simulink model "original_decfir"  (R2012b)
settings: Solver=FixedStepDiscrete  SolverMode=SingleTasking  StartTime=0.0  StopTime=5000  FixedStep=1  RelTol=1e-3
libraries: xbsIndex_r4 x1499, xps_library x1, casper_library_misc x1
(part 7 of 15)

== system original_decfir/dec_fir/fir_dbl_col6 ==
  real1 : Inport
  imag1 : Inport  Port=2
  real2 : Inport  Port=3
  imag2 : Inport  Port=4
  real3 : Inport  Port=5
  imag3 : Inport  Port=6
  real4 : Inport  Port=7
  imag4 : Inport  Port=8
  real5 : Inport  Port=9
  imag5 : Inport  Port=10
  real6 : Inport  Port=11
  imag6 : Inport  Port=12
  real7 : Inport  Port=13
  imag7 : Inport  Port=14
  real8 : Inport  Port=15
  imag8 : Inport  Port=16
  real_back1 : Inport  Port=17
  imag_back1 : Inport  Port=18
  real_back2 : Inport  Port=19
  imag_back2 : Inport  Port=20
  real_back3 : Inport  Port=21
  imag_back3 : Inport  Port=22
  real_back4 : Inport  Port=23
  imag_back4 : Inport  Port=24
  real_back5 : Inport  Port=25
  imag_back5 : Inport  Port=26
  real_back6 : Inport  Port=27
  imag_back6 : Inport  Port=28
  real_back7 : Inport  Port=29
  imag_back7 : Inport  Port=30
  real_back8 : Inport  Port=31
  imag_back8 : Inport  Port=32
  adder_tree1 : Subsystem  AncestorBlock=casper_library_misc/adder_tree  mask(adder_tree){n_inputs=8, latency=1, adder_imp=Behavioral, first_stage_hdl=off}
      mask prompts: n_inputs "Number of Inputs"; latency "Add Latency"; adder_imp "Adder implementation"; first_stage_hdl "Use behavioural HDL for first stage of adders"
      mask help:
      | Sums all inputs using a tree of adds and delays.
      |
      | Number of inputs: The number of inputs to the block to be summed
      | Add latency: The number of clock cycles to perform one addition (affects timing)..
      | Adder implementation: choice of fabric or DSP48E core, or behavioral HDL
      | Use behavioural HDL for first stage of adders: Causes the first stage of adders to be absorbed into DSP blocks if multipliers precede them (Virtex 5). Overrides Adder implementation
      mask init:
      | adder_tree_init(gcb, ...
      |     'n_inputs', n_inputs, ...
      |     'latency', latency, ...
      |     'adder_imp', adder_imp, ...
      |     'first_stage_hdl', first_stage_hdl);
      settings: AttributesFormatString=latency 3
      mask Help: eval('xlWeb(''http://casper.berkeley.edu/wiki/Adder_tree'')')
      mask TypeOptions adder_imp: Behavioral | Fabric | DSP48
  adder_tree2 : Subsystem  AncestorBlock=casper_library_misc/adder_tree  mask(adder_tree){n_inputs=8, latency=1, adder_imp=Behavioral, first_stage_hdl=off}
      mask prompts: n_inputs "Number of Inputs"; latency "Add Latency"; adder_imp "Adder implementation"; first_stage_hdl "Use behavioural HDL for first stage of adders"
      mask help:
      | Sums all inputs using a tree of adds and delays.
      |
      | Number of inputs: The number of inputs to the block to be summed
      | Add latency: The number of clock cycles to perform one addition (affects timing)..
      | Adder implementation: choice of fabric or DSP48E core, or behavioral HDL
      | Use behavioural HDL for first stage of adders: Causes the first stage of adders to be absorbed into DSP blocks if multipliers precede them (Virtex 5). Overrides Adder implementation
      mask init:
      | adder_tree_init(gcb, ...
      |     'n_inputs', n_inputs, ...
      |     'latency', latency, ...
      |     'adder_imp', adder_imp, ...
      |     'first_stage_hdl', first_stage_hdl);
      settings: AttributesFormatString=latency 3
      mask Help: eval('xlWeb(''http://casper.berkeley.edu/wiki/Adder_tree'')')
      mask TypeOptions adder_imp: Behavioral | Fabric | DSP48
  c1 : xbsIndex_r4/Constant  const=1  gui_display_data_type=Fixed-point  arith_type=Signed (2's comp)  n_bits=16  bin_pt=14  preci_type=Single  exp_width=8  frac_width=24  explicit_period=on  period=1  equ=P=C  opselect=C  inp2=PCIN>>17  opr=+  inp1=P  carry=CIN  dbl_ovrd=off  block_type=constant
  c2 : xbsIndex_r4/Constant  const=1  gui_display_data_type=Fixed-point  arith_type=Signed (2's comp)  n_bits=16  bin_pt=14  preci_type=Single  exp_width=8  frac_width=24  explicit_period=on  period=1  equ=P=C  opselect=C  inp2=PCIN>>17  opr=+  inp1=P  carry=CIN  dbl_ovrd=off  block_type=constant
  fir_dbl_tap1 : Subsystem  AncestorBlock=casper_library_downconverter/fir_dbl_tap  mask(fir_dbl_tap){factor=-0.0012722, add_latency=add_latency, mult_latency=mult_latency, coeff_bit_width=coeff_bit_width, coeff_bin_pt=coeff_bin_pt}
      mask prompts: add_latency "Add latency"; mult_latency "Mult latency"; coeff_bit_width "Coefficient bit width"; coeff_bin_pt "Coefficient binary point"
      mask init: same as original_decfir/dec_fir/fir_dbl_col1/fir_dbl_tap1
      mask Help: eval('xlWeb(''http://casper.berkeley.edu/wiki/Fir_dbl_tap'')')
  fir_dbl_tap2 : Subsystem  AncestorBlock=casper_library_downconverter/fir_dbl_tap  mask(fir_dbl_tap){factor=-0.0012742, add_latency=add_latency, mult_latency=mult_latency, coeff_bit_width=coeff_bit_width, coeff_bin_pt=coeff_bin_pt}
      mask prompts: add_latency "Add latency"; mult_latency "Mult latency"; coeff_bit_width "Coefficient bit width"; coeff_bin_pt "Coefficient binary point"
      mask init: same as original_decfir/dec_fir/fir_dbl_col1/fir_dbl_tap1
      mask Help: eval('xlWeb(''http://casper.berkeley.edu/wiki/Fir_dbl_tap'')')
  fir_dbl_tap3 : Subsystem  AncestorBlock=casper_library_downconverter/fir_dbl_tap  mask(fir_dbl_tap){factor=-0.0011107, add_latency=add_latency, mult_latency=mult_latency, coeff_bit_width=coeff_bit_width, coeff_bin_pt=coeff_bin_pt}
      mask prompts: add_latency "Add latency"; mult_latency "Mult latency"; coeff_bit_width "Coefficient bit width"; coeff_bin_pt "Coefficient binary point"
      mask init: same as original_decfir/dec_fir/fir_dbl_col1/fir_dbl_tap1
      mask Help: eval('xlWeb(''http://casper.berkeley.edu/wiki/Fir_dbl_tap'')')
  fir_dbl_tap4 : Subsystem  AncestorBlock=casper_library_downconverter/fir_dbl_tap  mask(fir_dbl_tap){factor=-0.00081658, add_latency=add_latency, mult_latency=mult_latency, coeff_bit_width=coeff_bit_width, coeff_bin_pt=coeff_bin_pt}
      mask prompts: add_latency "Add latency"; mult_latency "Mult latency"; coeff_bit_width "Coefficient bit width"; coeff_bin_pt "Coefficient binary point"
      mask init: same as original_decfir/dec_fir/fir_dbl_col1/fir_dbl_tap1
      mask Help: eval('xlWeb(''http://casper.berkeley.edu/wiki/Fir_dbl_tap'')')
  fir_dbl_tap5 : Subsystem  AncestorBlock=casper_library_downconverter/fir_dbl_tap  mask(fir_dbl_tap){factor=-0.0004409, add_latency=add_latency, mult_latency=mult_latency, coeff_bit_width=coeff_bit_width, coeff_bin_pt=coeff_bin_pt}
      mask prompts: add_latency "Add latency"; mult_latency "Mult latency"; coeff_bit_width "Coefficient bit width"; coeff_bin_pt "Coefficient binary point"
      mask init: same as original_decfir/dec_fir/fir_dbl_col1/fir_dbl_tap1
      mask Help: eval('xlWeb(''http://casper.berkeley.edu/wiki/Fir_dbl_tap'')')
  fir_dbl_tap6 : Subsystem  AncestorBlock=casper_library_downconverter/fir_dbl_tap  mask(fir_dbl_tap){factor=-3.9415e-05, add_latency=add_latency, mult_latency=mult_latency, coeff_bit_width=coeff_bit_width, coeff_bin_pt=coeff_bin_pt}
      mask prompts: add_latency "Add latency"; mult_latency "Mult latency"; coeff_bit_width "Coefficient bit width"; coeff_bin_pt "Coefficient binary point"
      mask init: same as original_decfir/dec_fir/fir_dbl_col1/fir_dbl_tap1
      mask Help: eval('xlWeb(''http://casper.berkeley.edu/wiki/Fir_dbl_tap'')')
  fir_dbl_tap7 : Subsystem  AncestorBlock=casper_library_downconverter/fir_dbl_tap  mask(fir_dbl_tap){factor=0.00033331, add_latency=add_latency, mult_latency=mult_latency, coeff_bit_width=coeff_bit_width, coeff_bin_pt=coeff_bin_pt}
      mask prompts: add_latency "Add latency"; mult_latency "Mult latency"; coeff_bit_width "Coefficient bit width"; coeff_bin_pt "Coefficient binary point"
      mask init: same as original_decfir/dec_fir/fir_dbl_col1/fir_dbl_tap1
      mask Help: eval('xlWeb(''http://casper.berkeley.edu/wiki/Fir_dbl_tap'')')
  fir_dbl_tap8 : Subsystem  AncestorBlock=casper_library_downconverter/fir_dbl_tap  mask(fir_dbl_tap){factor=0.00063107, add_latency=add_latency, mult_latency=mult_latency, coeff_bit_width=coeff_bit_width, coeff_bin_pt=coeff_bin_pt}
      mask prompts: add_latency "Add latency"; mult_latency "Mult latency"; coeff_bit_width "Coefficient bit width"; coeff_bin_pt "Coefficient binary point"
      mask init: same as original_decfir/dec_fir/fir_dbl_col1/fir_dbl_tap1
      mask Help: eval('xlWeb(''http://casper.berkeley.edu/wiki/Fir_dbl_tap'')')
  term1 : Terminator
  term2 : Terminator
  real_out1 : Outport
  imag_out1 : Outport  Port=2
  real_out2 : Outport  Port=3
  imag_out2 : Outport  Port=4
  real_out3 : Outport  Port=5
  imag_out3 : Outport  Port=6
  real_out4 : Outport  Port=7
  imag_out4 : Outport  Port=8
  real_out5 : Outport  Port=9
  imag_out5 : Outport  Port=10
  real_out6 : Outport  Port=11
  imag_out6 : Outport  Port=12
  real_out7 : Outport  Port=13
  imag_out7 : Outport  Port=14
  real_out8 : Outport  Port=15
  imag_out8 : Outport  Port=16
  real_back_out1 : Outport  Port=17
  imag_back_out1 : Outport  Port=18
  real_back_out2 : Outport  Port=19
  imag_back_out2 : Outport  Port=20
  real_back_out3 : Outport  Port=21
  imag_back_out3 : Outport  Port=22
  real_back_out4 : Outport  Port=23
  imag_back_out4 : Outport  Port=24
  real_back_out5 : Outport  Port=25
  imag_back_out5 : Outport  Port=26
  real_back_out6 : Outport  Port=27
  imag_back_out6 : Outport  Port=28
  real_back_out7 : Outport  Port=29
  imag_back_out7 : Outport  Port=30
  real_back_out8 : Outport  Port=31
  imag_back_out8 : Outport  Port=32
  real_sum : Outport  Port=33
  imag_sum : Outport  Port=34
  wires:
  adder_tree1/1(sync_out) -> term1/1
  adder_tree2/1(sync_out) -> term2/1
  c1/1 -> adder_tree1/1(sync)
  c2/1 -> adder_tree2/1(sync)
  adder_tree1/2(dout) -> real_sum/1
  adder_tree2/2(dout) -> imag_sum/1
  real1/1 -> fir_dbl_tap1/1(a)
  imag1/1 -> fir_dbl_tap1/2(b)
  real_back8/1 -> fir_dbl_tap1/3(c)
  imag_back8/1 -> fir_dbl_tap1/4(d)
  fir_dbl_tap1/1(a_out) -> real_out1/1
  fir_dbl_tap1/2(b_out) -> imag_out1/1
  fir_dbl_tap1/3(c_out) -> real_back_out8/1
  fir_dbl_tap1/4(d_out) -> imag_back_out8/1
  fir_dbl_tap1/5(real) -> adder_tree1/2(din1)
  fir_dbl_tap1/6(imag) -> adder_tree2/2(din1)
  real2/1 -> fir_dbl_tap2/1(a)
  imag2/1 -> fir_dbl_tap2/2(b)
  real_back7/1 -> fir_dbl_tap2/3(c)
  imag_back7/1 -> fir_dbl_tap2/4(d)
  fir_dbl_tap2/1(a_out) -> real_out2/1
  fir_dbl_tap2/2(b_out) -> imag_out2/1
  fir_dbl_tap2/3(c_out) -> real_back_out7/1
  fir_dbl_tap2/4(d_out) -> imag_back_out7/1
  fir_dbl_tap2/5(real) -> adder_tree1/3(din2)
  fir_dbl_tap2/6(imag) -> adder_tree2/3(din2)
  real3/1 -> fir_dbl_tap3/1(a)
  imag3/1 -> fir_dbl_tap3/2(b)
  real_back6/1 -> fir_dbl_tap3/3(c)
  imag_back6/1 -> fir_dbl_tap3/4(d)
  fir_dbl_tap3/1(a_out) -> real_out3/1
  fir_dbl_tap3/2(b_out) -> imag_out3/1
  fir_dbl_tap3/3(c_out) -> real_back_out6/1
  fir_dbl_tap3/4(d_out) -> imag_back_out6/1
  fir_dbl_tap3/5(real) -> adder_tree1/4(din3)
  fir_dbl_tap3/6(imag) -> adder_tree2/4(din3)
  real4/1 -> fir_dbl_tap4/1(a)
  imag4/1 -> fir_dbl_tap4/2(b)
  real_back5/1 -> fir_dbl_tap4/3(c)
  imag_back5/1 -> fir_dbl_tap4/4(d)
  fir_dbl_tap4/1(a_out) -> real_out4/1
  fir_dbl_tap4/2(b_out) -> imag_out4/1
  fir_dbl_tap4/3(c_out) -> real_back_out5/1
  fir_dbl_tap4/4(d_out) -> imag_back_out5/1
  fir_dbl_tap4/5(real) -> adder_tree1/5(din4)
  fir_dbl_tap4/6(imag) -> adder_tree2/5(din4)
  real5/1 -> fir_dbl_tap5/1(a)
  imag5/1 -> fir_dbl_tap5/2(b)
  real_back4/1 -> fir_dbl_tap5/3(c)
  imag_back4/1 -> fir_dbl_tap5/4(d)
  fir_dbl_tap5/1(a_out) -> real_out5/1
  fir_dbl_tap5/2(b_out) -> imag_out5/1
  fir_dbl_tap5/3(c_out) -> real_back_out4/1
  fir_dbl_tap5/4(d_out) -> imag_back_out4/1
  fir_dbl_tap5/5(real) -> adder_tree1/6(din5)
  fir_dbl_tap5/6(imag) -> adder_tree2/6(din5)
  real6/1 -> fir_dbl_tap6/1(a)
  imag6/1 -> fir_dbl_tap6/2(b)
  real_back3/1 -> fir_dbl_tap6/3(c)
  imag_back3/1 -> fir_dbl_tap6/4(d)
  fir_dbl_tap6/1(a_out) -> real_out6/1
  fir_dbl_tap6/2(b_out) -> imag_out6/1
  fir_dbl_tap6/3(c_out) -> real_back_out3/1
  fir_dbl_tap6/4(d_out) -> imag_back_out3/1
  fir_dbl_tap6/5(real) -> adder_tree1/7(din6)
  fir_dbl_tap6/6(imag) -> adder_tree2/7(din6)
  real7/1 -> fir_dbl_tap7/1(a)
  imag7/1 -> fir_dbl_tap7/2(b)
  real_back2/1 -> fir_dbl_tap7/3(c)
  imag_back2/1 -> fir_dbl_tap7/4(d)
  fir_dbl_tap7/1(a_out) -> real_out7/1
  fir_dbl_tap7/2(b_out) -> imag_out7/1
  fir_dbl_tap7/3(c_out) -> real_back_out2/1
  fir_dbl_tap7/4(d_out) -> imag_back_out2/1
  fir_dbl_tap7/5(real) -> adder_tree1/8(din7)
  fir_dbl_tap7/6(imag) -> adder_tree2/8(din7)
  real8/1 -> fir_dbl_tap8/1(a)
  imag8/1 -> fir_dbl_tap8/2(b)
  real_back1/1 -> fir_dbl_tap8/3(c)
  imag_back1/1 -> fir_dbl_tap8/4(d)
  fir_dbl_tap8/1(a_out) -> real_out8/1
  fir_dbl_tap8/2(b_out) -> imag_out8/1
  fir_dbl_tap8/3(c_out) -> real_back_out1/1
  fir_dbl_tap8/4(d_out) -> imag_back_out1/1
  fir_dbl_tap8/5(real) -> adder_tree1/9(din8)
  fir_dbl_tap8/6(imag) -> adder_tree2/9(din8)

== system original_decfir/dec_fir/fir_dbl_col7 ==
  real1 : Inport
  imag1 : Inport  Port=2
  real2 : Inport  Port=3
  imag2 : Inport  Port=4
  real3 : Inport  Port=5
  imag3 : Inport  Port=6
  real4 : Inport  Port=7
  imag4 : Inport  Port=8
  real5 : Inport  Port=9
  imag5 : Inport  Port=10
  real6 : Inport  Port=11
  imag6 : Inport  Port=12
  real7 : Inport  Port=13
  imag7 : Inport  Port=14
  real8 : Inport  Port=15
  imag8 : Inport  Port=16
  real_back1 : Inport  Port=17
  imag_back1 : Inport  Port=18
  real_back2 : Inport  Port=19
  imag_back2 : Inport  Port=20
  real_back3 : Inport  Port=21
  imag_back3 : Inport  Port=22
  real_back4 : Inport  Port=23
  imag_back4 : Inport  Port=24
  real_back5 : Inport  Port=25
  imag_back5 : Inport  Port=26
  real_back6 : Inport  Port=27
  imag_back6 : Inport  Port=28
  real_back7 : Inport  Port=29
  imag_back7 : Inport  Port=30
  real_back8 : Inport  Port=31
  imag_back8 : Inport  Port=32
  adder_tree1 : Subsystem  AncestorBlock=casper_library_misc/adder_tree  mask(adder_tree){n_inputs=8, latency=1, adder_imp=Behavioral, first_stage_hdl=off}
      mask prompts: n_inputs "Number of Inputs"; latency "Add Latency"; adder_imp "Adder implementation"; first_stage_hdl "Use behavioural HDL for first stage of adders"
      mask help:
      | Sums all inputs using a tree of adds and delays.
      |
      | Number of inputs: The number of inputs to the block to be summed
      | Add latency: The number of clock cycles to perform one addition (affects timing)..
      | Adder implementation: choice of fabric or DSP48E core, or behavioral HDL
      | Use behavioural HDL for first stage of adders: Causes the first stage of adders to be absorbed into DSP blocks if multipliers precede them (Virtex 5). Overrides Adder implementation
      mask init:
      | adder_tree_init(gcb, ...
      |     'n_inputs', n_inputs, ...
      |     'latency', latency, ...
      |     'adder_imp', adder_imp, ...
      |     'first_stage_hdl', first_stage_hdl);
      settings: AttributesFormatString=latency 3
      mask Help: eval('xlWeb(''http://casper.berkeley.edu/wiki/Adder_tree'')')
      mask TypeOptions adder_imp: Behavioral | Fabric | DSP48
  adder_tree2 : Subsystem  AncestorBlock=casper_library_misc/adder_tree  mask(adder_tree){n_inputs=8, latency=1, adder_imp=Behavioral, first_stage_hdl=off}
      mask prompts: n_inputs "Number of Inputs"; latency "Add Latency"; adder_imp "Adder implementation"; first_stage_hdl "Use behavioural HDL for first stage of adders"
      mask help:
      | Sums all inputs using a tree of adds and delays.
      |
      | Number of inputs: The number of inputs to the block to be summed
      | Add latency: The number of clock cycles to perform one addition (affects timing)..
      | Adder implementation: choice of fabric or DSP48E core, or behavioral HDL
      | Use behavioural HDL for first stage of adders: Causes the first stage of adders to be absorbed into DSP blocks if multipliers precede them (Virtex 5). Overrides Adder implementation
      mask init:
      | adder_tree_init(gcb, ...
      |     'n_inputs', n_inputs, ...
      |     'latency', latency, ...
      |     'adder_imp', adder_imp, ...
      |     'first_stage_hdl', first_stage_hdl);
      settings: AttributesFormatString=latency 3
      mask Help: eval('xlWeb(''http://casper.berkeley.edu/wiki/Adder_tree'')')
      mask TypeOptions adder_imp: Behavioral | Fabric | DSP48
  c1 : xbsIndex_r4/Constant  const=1  gui_display_data_type=Fixed-point  arith_type=Signed (2's comp)  n_bits=16  bin_pt=14  preci_type=Single  exp_width=8  frac_width=24  explicit_period=on  period=1  equ=P=C  opselect=C  inp2=PCIN>>17  opr=+  inp1=P  carry=CIN  dbl_ovrd=off  block_type=constant
  c2 : xbsIndex_r4/Constant  const=1  gui_display_data_type=Fixed-point  arith_type=Signed (2's comp)  n_bits=16  bin_pt=14  preci_type=Single  exp_width=8  frac_width=24  explicit_period=on  period=1  equ=P=C  opselect=C  inp2=PCIN>>17  opr=+  inp1=P  carry=CIN  dbl_ovrd=off  block_type=constant
  fir_dbl_tap1 : Subsystem  AncestorBlock=casper_library_downconverter/fir_dbl_tap  mask(fir_dbl_tap){factor=0.0018361, add_latency=add_latency, mult_latency=mult_latency, coeff_bit_width=coeff_bit_width, coeff_bin_pt=coeff_bin_pt}
      mask prompts: add_latency "Add latency"; mult_latency "Mult latency"; coeff_bit_width "Coefficient bit width"; coeff_bin_pt "Coefficient binary point"
      mask init: same as original_decfir/dec_fir/fir_dbl_col1/fir_dbl_tap1
      mask Help: eval('xlWeb(''http://casper.berkeley.edu/wiki/Fir_dbl_tap'')')
  fir_dbl_tap2 : Subsystem  AncestorBlock=casper_library_downconverter/fir_dbl_tap  mask(fir_dbl_tap){factor=0.0017079, add_latency=add_latency, mult_latency=mult_latency, coeff_bit_width=coeff_bit_width, coeff_bin_pt=coeff_bin_pt}
      mask prompts: add_latency "Add latency"; mult_latency "Mult latency"; coeff_bit_width "Coefficient bit width"; coeff_bin_pt "Coefficient binary point"
      mask init: same as original_decfir/dec_fir/fir_dbl_col1/fir_dbl_tap1
      mask Help: eval('xlWeb(''http://casper.berkeley.edu/wiki/Fir_dbl_tap'')')
  fir_dbl_tap3 : Subsystem  AncestorBlock=casper_library_downconverter/fir_dbl_tap  mask(fir_dbl_tap){factor=0.0013679, add_latency=add_latency, mult_latency=mult_latency, coeff_bit_width=coeff_bit_width, coeff_bin_pt=coeff_bin_pt}
      mask prompts: add_latency "Add latency"; mult_latency "Mult latency"; coeff_bit_width "Coefficient bit width"; coeff_bin_pt "Coefficient binary point"
      mask init: same as original_decfir/dec_fir/fir_dbl_col1/fir_dbl_tap1
      mask Help: eval('xlWeb(''http://casper.berkeley.edu/wiki/Fir_dbl_tap'')')
  fir_dbl_tap4 : Subsystem  AncestorBlock=casper_library_downconverter/fir_dbl_tap  mask(fir_dbl_tap){factor=0.00087646, add_latency=add_latency, mult_latency=mult_latency, coeff_bit_width=coeff_bit_width, coeff_bin_pt=coeff_bin_pt}
      mask prompts: add_latency "Add latency"; mult_latency "Mult latency"; coeff_bit_width "Coefficient bit width"; coeff_bin_pt "Coefficient binary point"
      mask init: same as original_decfir/dec_fir/fir_dbl_col1/fir_dbl_tap1
      mask Help: eval('xlWeb(''http://casper.berkeley.edu/wiki/Fir_dbl_tap'')')
  fir_dbl_tap5 : Subsystem  AncestorBlock=casper_library_downconverter/fir_dbl_tap  mask(fir_dbl_tap){factor=0.00030942, add_latency=add_latency, mult_latency=mult_latency, coeff_bit_width=coeff_bit_width, coeff_bin_pt=coeff_bin_pt}
      mask prompts: add_latency "Add latency"; mult_latency "Mult latency"; coeff_bit_width "Coefficient bit width"; coeff_bin_pt "Coefficient binary point"
      mask init: same as original_decfir/dec_fir/fir_dbl_col1/fir_dbl_tap1
      mask Help: eval('xlWeb(''http://casper.berkeley.edu/wiki/Fir_dbl_tap'')')
  fir_dbl_tap6 : Subsystem  AncestorBlock=casper_library_downconverter/fir_dbl_tap  mask(fir_dbl_tap){factor=-0.00025349, add_latency=add_latency, mult_latency=mult_latency, coeff_bit_width=coeff_bit_width, coeff_bin_pt=coeff_bin_pt}
      mask prompts: add_latency "Add latency"; mult_latency "Mult latency"; coeff_bit_width "Coefficient bit width"; coeff_bin_pt "Coefficient binary point"
      mask init: same as original_decfir/dec_fir/fir_dbl_col1/fir_dbl_tap1
      mask Help: eval('xlWeb(''http://casper.berkeley.edu/wiki/Fir_dbl_tap'')')
  fir_dbl_tap7 : Subsystem  AncestorBlock=casper_library_downconverter/fir_dbl_tap  mask(fir_dbl_tap){factor=-0.0007392, add_latency=add_latency, mult_latency=mult_latency, coeff_bit_width=coeff_bit_width, coeff_bin_pt=coeff_bin_pt}
      mask prompts: add_latency "Add latency"; mult_latency "Mult latency"; coeff_bit_width "Coefficient bit width"; coeff_bin_pt "Coefficient binary point"
      mask init: same as original_decfir/dec_fir/fir_dbl_col1/fir_dbl_tap1
      mask Help: eval('xlWeb(''http://casper.berkeley.edu/wiki/Fir_dbl_tap'')')
  fir_dbl_tap8 : Subsystem  AncestorBlock=casper_library_downconverter/fir_dbl_tap  mask(fir_dbl_tap){factor=-0.0010905, add_latency=add_latency, mult_latency=mult_latency, coeff_bit_width=coeff_bit_width, coeff_bin_pt=coeff_bin_pt}
      mask prompts: add_latency "Add latency"; mult_latency "Mult latency"; coeff_bit_width "Coefficient bit width"; coeff_bin_pt "Coefficient binary point"
      mask init: same as original_decfir/dec_fir/fir_dbl_col1/fir_dbl_tap1
      mask Help: eval('xlWeb(''http://casper.berkeley.edu/wiki/Fir_dbl_tap'')')
  term1 : Terminator
  term2 : Terminator
  real_out1 : Outport
  imag_out1 : Outport  Port=2
  real_out2 : Outport  Port=3
  imag_out2 : Outport  Port=4
  real_out3 : Outport  Port=5
  imag_out3 : Outport  Port=6
  real_out4 : Outport  Port=7
  imag_out4 : Outport  Port=8
  real_out5 : Outport  Port=9
  imag_out5 : Outport  Port=10
  real_out6 : Outport  Port=11
  imag_out6 : Outport  Port=12
  real_out7 : Outport  Port=13
  imag_out7 : Outport  Port=14
  real_out8 : Outport  Port=15
  imag_out8 : Outport  Port=16
  real_back_out1 : Outport  Port=17
  imag_back_out1 : Outport  Port=18
  real_back_out2 : Outport  Port=19
  imag_back_out2 : Outport  Port=20
  real_back_out3 : Outport  Port=21
  imag_back_out3 : Outport  Port=22
  real_back_out4 : Outport  Port=23
  imag_back_out4 : Outport  Port=24
  real_back_out5 : Outport  Port=25
  imag_back_out5 : Outport  Port=26
  real_back_out6 : Outport  Port=27
  imag_back_out6 : Outport  Port=28
  real_back_out7 : Outport  Port=29
  imag_back_out7 : Outport  Port=30
  real_back_out8 : Outport  Port=31
  imag_back_out8 : Outport  Port=32
  real_sum : Outport  Port=33
  imag_sum : Outport  Port=34
  wires:
  adder_tree1/1(sync_out) -> term1/1
  adder_tree2/1(sync_out) -> term2/1
  c1/1 -> adder_tree1/1(sync)
  c2/1 -> adder_tree2/1(sync)
  adder_tree1/2(dout) -> real_sum/1
  adder_tree2/2(dout) -> imag_sum/1
  real1/1 -> fir_dbl_tap1/1(a)
  imag1/1 -> fir_dbl_tap1/2(b)
  real_back8/1 -> fir_dbl_tap1/3(c)
  imag_back8/1 -> fir_dbl_tap1/4(d)
  fir_dbl_tap1/1(a_out) -> real_out1/1
  fir_dbl_tap1/2(b_out) -> imag_out1/1
  fir_dbl_tap1/3(c_out) -> real_back_out8/1
  fir_dbl_tap1/4(d_out) -> imag_back_out8/1
  fir_dbl_tap1/5(real) -> adder_tree1/2(din1)
  fir_dbl_tap1/6(imag) -> adder_tree2/2(din1)
  real2/1 -> fir_dbl_tap2/1(a)
  imag2/1 -> fir_dbl_tap2/2(b)
  real_back7/1 -> fir_dbl_tap2/3(c)
  imag_back7/1 -> fir_dbl_tap2/4(d)
  fir_dbl_tap2/1(a_out) -> real_out2/1
  fir_dbl_tap2/2(b_out) -> imag_out2/1
  fir_dbl_tap2/3(c_out) -> real_back_out7/1
  fir_dbl_tap2/4(d_out) -> imag_back_out7/1
  fir_dbl_tap2/5(real) -> adder_tree1/3(din2)
  fir_dbl_tap2/6(imag) -> adder_tree2/3(din2)
  real3/1 -> fir_dbl_tap3/1(a)
  imag3/1 -> fir_dbl_tap3/2(b)
  real_back6/1 -> fir_dbl_tap3/3(c)
  imag_back6/1 -> fir_dbl_tap3/4(d)
  fir_dbl_tap3/1(a_out) -> real_out3/1
  fir_dbl_tap3/2(b_out) -> imag_out3/1
  fir_dbl_tap3/3(c_out) -> real_back_out6/1
  fir_dbl_tap3/4(d_out) -> imag_back_out6/1
  fir_dbl_tap3/5(real) -> adder_tree1/4(din3)
  fir_dbl_tap3/6(imag) -> adder_tree2/4(din3)
  real4/1 -> fir_dbl_tap4/1(a)
  imag4/1 -> fir_dbl_tap4/2(b)
  real_back5/1 -> fir_dbl_tap4/3(c)
  imag_back5/1 -> fir_dbl_tap4/4(d)
  fir_dbl_tap4/1(a_out) -> real_out4/1
  fir_dbl_tap4/2(b_out) -> imag_out4/1
  fir_dbl_tap4/3(c_out) -> real_back_out5/1
  fir_dbl_tap4/4(d_out) -> imag_back_out5/1
  fir_dbl_tap4/5(real) -> adder_tree1/5(din4)
  fir_dbl_tap4/6(imag) -> adder_tree2/5(din4)
  real5/1 -> fir_dbl_tap5/1(a)
  imag5/1 -> fir_dbl_tap5/2(b)
  real_back4/1 -> fir_dbl_tap5/3(c)
  imag_back4/1 -> fir_dbl_tap5/4(d)
  fir_dbl_tap5/1(a_out) -> real_out5/1
  fir_dbl_tap5/2(b_out) -> imag_out5/1
  fir_dbl_tap5/3(c_out) -> real_back_out4/1
  fir_dbl_tap5/4(d_out) -> imag_back_out4/1
  fir_dbl_tap5/5(real) -> adder_tree1/6(din5)
  fir_dbl_tap5/6(imag) -> adder_tree2/6(din5)
  real6/1 -> fir_dbl_tap6/1(a)
  imag6/1 -> fir_dbl_tap6/2(b)
  real_back3/1 -> fir_dbl_tap6/3(c)
  imag_back3/1 -> fir_dbl_tap6/4(d)
  fir_dbl_tap6/1(a_out) -> real_out6/1
  fir_dbl_tap6/2(b_out) -> imag_out6/1
  fir_dbl_tap6/3(c_out) -> real_back_out3/1
  fir_dbl_tap6/4(d_out) -> imag_back_out3/1
  fir_dbl_tap6/5(real) -> adder_tree1/7(din6)
  fir_dbl_tap6/6(imag) -> adder_tree2/7(din6)
  real7/1 -> fir_dbl_tap7/1(a)
  imag7/1 -> fir_dbl_tap7/2(b)
  real_back2/1 -> fir_dbl_tap7/3(c)
  imag_back2/1 -> fir_dbl_tap7/4(d)
  fir_dbl_tap7/1(a_out) -> real_out7/1
  fir_dbl_tap7/2(b_out) -> imag_out7/1
  fir_dbl_tap7/3(c_out) -> real_back_out2/1
  fir_dbl_tap7/4(d_out) -> imag_back_out2/1
  fir_dbl_tap7/5(real) -> adder_tree1/8(din7)
  fir_dbl_tap7/6(imag) -> adder_tree2/8(din7)
  real8/1 -> fir_dbl_tap8/1(a)
  imag8/1 -> fir_dbl_tap8/2(b)
  real_back1/1 -> fir_dbl_tap8/3(c)
  imag_back1/1 -> fir_dbl_tap8/4(d)
  fir_dbl_tap8/1(a_out) -> real_out8/1
  fir_dbl_tap8/2(b_out) -> imag_out8/1
  fir_dbl_tap8/3(c_out) -> real_back_out1/1
  fir_dbl_tap8/4(d_out) -> imag_back_out1/1
  fir_dbl_tap8/5(real) -> adder_tree1/9(din8)
  fir_dbl_tap8/6(imag) -> adder_tree2/9(din8)

== system original_decfir/dec_fir/fir_dbl_col8 ==
  real1 : Inport
  imag1 : Inport  Port=2
  real2 : Inport  Port=3
  imag2 : Inport  Port=4
  real3 : Inport  Port=5
  imag3 : Inport  Port=6
  real4 : Inport  Port=7
  imag4 : Inport  Port=8
  real5 : Inport  Port=9
  imag5 : Inport  Port=10
  real6 : Inport  Port=11
  imag6 : Inport  Port=12
  real7 : Inport  Port=13
  imag7 : Inport  Port=14
  real8 : Inport  Port=15
  imag8 : Inport  Port=16
  real_back1 : Inport  Port=17
  imag_back1 : Inport  Port=18
  real_back2 : Inport  Port=19
  imag_back2 : Inport  Port=20
  real_back3 : Inport  Port=21
  imag_back3 : Inport  Port=22
  real_back4 : Inport  Port=23
  imag_back4 : Inport  Port=24
  real_back5 : Inport  Port=25
  imag_back5 : Inport  Port=26
  real_back6 : Inport  Port=27
  imag_back6 : Inport  Port=28
  real_back7 : Inport  Port=29
  imag_back7 : Inport  Port=30
  real_back8 : Inport  Port=31
  imag_back8 : Inport  Port=32
  adder_tree1 : Subsystem  AncestorBlock=casper_library_misc/adder_tree  mask(adder_tree){n_inputs=8, latency=1, adder_imp=Behavioral, first_stage_hdl=off}
      mask prompts: n_inputs "Number of Inputs"; latency "Add Latency"; adder_imp "Adder implementation"; first_stage_hdl "Use behavioural HDL for first stage of adders"
      mask help:
      | Sums all inputs using a tree of adds and delays.
      |
      | Number of inputs: The number of inputs to the block to be summed
      | Add latency: The number of clock cycles to perform one addition (affects timing)..
      | Adder implementation: choice of fabric or DSP48E core, or behavioral HDL
      | Use behavioural HDL for first stage of adders: Causes the first stage of adders to be absorbed into DSP blocks if multipliers precede them (Virtex 5). Overrides Adder implementation
      mask init:
      | adder_tree_init(gcb, ...
      |     'n_inputs', n_inputs, ...
      |     'latency', latency, ...
      |     'adder_imp', adder_imp, ...
      |     'first_stage_hdl', first_stage_hdl);
      settings: AttributesFormatString=latency 3
      mask Help: eval('xlWeb(''http://casper.berkeley.edu/wiki/Adder_tree'')')
      mask TypeOptions adder_imp: Behavioral | Fabric | DSP48
  adder_tree2 : Subsystem  AncestorBlock=casper_library_misc/adder_tree  mask(adder_tree){n_inputs=8, latency=1, adder_imp=Behavioral, first_stage_hdl=off}
      mask prompts: n_inputs "Number of Inputs"; latency "Add Latency"; adder_imp "Adder implementation"; first_stage_hdl "Use behavioural HDL for first stage of adders"
      mask help:
      | Sums all inputs using a tree of adds and delays.
      |
      | Number of inputs: The number of inputs to the block to be summed
      | Add latency: The number of clock cycles to perform one addition (affects timing)..
      | Adder implementation: choice of fabric or DSP48E core, or behavioral HDL
      | Use behavioural HDL for first stage of adders: Causes the first stage of adders to be absorbed into DSP blocks if multipliers precede them (Virtex 5). Overrides Adder implementation
      mask init:
      | adder_tree_init(gcb, ...
      |     'n_inputs', n_inputs, ...
      |     'latency', latency, ...
      |     'adder_imp', adder_imp, ...
      |     'first_stage_hdl', first_stage_hdl);
      settings: AttributesFormatString=latency 3
      mask Help: eval('xlWeb(''http://casper.berkeley.edu/wiki/Adder_tree'')')
      mask TypeOptions adder_imp: Behavioral | Fabric | DSP48
  c1 : xbsIndex_r4/Constant  const=1  gui_display_data_type=Fixed-point  arith_type=Signed (2's comp)  n_bits=16  bin_pt=14  preci_type=Single  exp_width=8  frac_width=24  explicit_period=on  period=1  equ=P=C  opselect=C  inp2=PCIN>>17  opr=+  inp1=P  carry=CIN  dbl_ovrd=off  block_type=constant
  c2 : xbsIndex_r4/Constant  const=1  gui_display_data_type=Fixed-point  arith_type=Signed (2's comp)  n_bits=16  bin_pt=14  preci_type=Single  exp_width=8  frac_width=24  explicit_period=on  period=1  equ=P=C  opselect=C  inp2=PCIN>>17  opr=+  inp1=P  carry=CIN  dbl_ovrd=off  block_type=constant
  fir_dbl_tap1 : Subsystem  AncestorBlock=casper_library_downconverter/fir_dbl_tap  mask(fir_dbl_tap){factor=-0.0024941, add_latency=add_latency, mult_latency=mult_latency, coeff_bit_width=coeff_bit_width, coeff_bin_pt=coeff_bin_pt}
      mask prompts: add_latency "Add latency"; mult_latency "Mult latency"; coeff_bit_width "Coefficient bit width"; coeff_bin_pt "Coefficient binary point"
      mask init: same as original_decfir/dec_fir/fir_dbl_col1/fir_dbl_tap1
      mask Help: eval('xlWeb(''http://casper.berkeley.edu/wiki/Fir_dbl_tap'')')
  fir_dbl_tap2 : Subsystem  AncestorBlock=casper_library_downconverter/fir_dbl_tap  mask(fir_dbl_tap){factor=-0.0021466, add_latency=add_latency, mult_latency=mult_latency, coeff_bit_width=coeff_bit_width, coeff_bin_pt=coeff_bin_pt}
      mask prompts: add_latency "Add latency"; mult_latency "Mult latency"; coeff_bit_width "Coefficient bit width"; coeff_bin_pt "Coefficient binary point"
      mask init: same as original_decfir/dec_fir/fir_dbl_col1/fir_dbl_tap1
      mask Help: eval('xlWeb(''http://casper.berkeley.edu/wiki/Fir_dbl_tap'')')
  fir_dbl_tap3 : Subsystem  AncestorBlock=casper_library_downconverter/fir_dbl_tap  mask(fir_dbl_tap){factor=-0.0015457, add_latency=add_latency, mult_latency=mult_latency, coeff_bit_width=coeff_bit_width, coeff_bin_pt=coeff_bin_pt}
      mask prompts: add_latency "Add latency"; mult_latency "Mult latency"; coeff_bit_width "Coefficient bit width"; coeff_bin_pt "Coefficient binary point"
      mask init: same as original_decfir/dec_fir/fir_dbl_col1/fir_dbl_tap1
      mask Help: eval('xlWeb(''http://casper.berkeley.edu/wiki/Fir_dbl_tap'')')
  fir_dbl_tap4 : Subsystem  AncestorBlock=casper_library_downconverter/fir_dbl_tap  mask(fir_dbl_tap){factor=-0.00078824, add_latency=add_latency, mult_latency=mult_latency, coeff_bit_width=coeff_bit_width, coeff_bin_pt=coeff_bin_pt}
      mask prompts: add_latency "Add latency"; mult_latency "Mult latency"; coeff_bit_width "Coefficient bit width"; coeff_bin_pt "Coefficient binary point"
      mask init: same as original_decfir/dec_fir/fir_dbl_col1/fir_dbl_tap1
      mask Help: eval('xlWeb(''http://casper.berkeley.edu/wiki/Fir_dbl_tap'')')
  fir_dbl_tap5 : Subsystem  AncestorBlock=casper_library_downconverter/fir_dbl_tap  mask(fir_dbl_tap){factor=1.582e-05, add_latency=add_latency, mult_latency=mult_latency, coeff_bit_width=coeff_bit_width, coeff_bin_pt=coeff_bin_pt}
      mask prompts: add_latency "Add latency"; mult_latency "Mult latency"; coeff_bit_width "Coefficient bit width"; coeff_bin_pt "Coefficient binary point"
      mask init: same as original_decfir/dec_fir/fir_dbl_col1/fir_dbl_tap1
      mask Help: eval('xlWeb(''http://casper.berkeley.edu/wiki/Fir_dbl_tap'')')
  fir_dbl_tap6 : Subsystem  AncestorBlock=casper_library_downconverter/fir_dbl_tap  mask(fir_dbl_tap){factor=0.00075832, add_latency=add_latency, mult_latency=mult_latency, coeff_bit_width=coeff_bit_width, coeff_bin_pt=coeff_bin_pt}
      mask prompts: add_latency "Add latency"; mult_latency "Mult latency"; coeff_bit_width "Coefficient bit width"; coeff_bin_pt "Coefficient binary point"
      mask init: same as original_decfir/dec_fir/fir_dbl_col1/fir_dbl_tap1
      mask Help: eval('xlWeb(''http://casper.berkeley.edu/wiki/Fir_dbl_tap'')')
  fir_dbl_tap7 : Subsystem  AncestorBlock=casper_library_downconverter/fir_dbl_tap  mask(fir_dbl_tap){factor=0.0013471, add_latency=add_latency, mult_latency=mult_latency, coeff_bit_width=coeff_bit_width, coeff_bin_pt=coeff_bin_pt}
      mask prompts: add_latency "Add latency"; mult_latency "Mult latency"; coeff_bit_width "Coefficient bit width"; coeff_bin_pt "Coefficient binary point"
      mask init: same as original_decfir/dec_fir/fir_dbl_col1/fir_dbl_tap1
      mask Help: eval('xlWeb(''http://casper.berkeley.edu/wiki/Fir_dbl_tap'')')
  fir_dbl_tap8 : Subsystem  AncestorBlock=casper_library_downconverter/fir_dbl_tap  mask(fir_dbl_tap){factor=0.001717, add_latency=add_latency, mult_latency=mult_latency, coeff_bit_width=coeff_bit_width, coeff_bin_pt=coeff_bin_pt}
      mask prompts: add_latency "Add latency"; mult_latency "Mult latency"; coeff_bit_width "Coefficient bit width"; coeff_bin_pt "Coefficient binary point"
      mask init: same as original_decfir/dec_fir/fir_dbl_col1/fir_dbl_tap1
      mask Help: eval('xlWeb(''http://casper.berkeley.edu/wiki/Fir_dbl_tap'')')
  term1 : Terminator
  term2 : Terminator
  real_out1 : Outport
  imag_out1 : Outport  Port=2
  real_out2 : Outport  Port=3
  imag_out2 : Outport  Port=4
  real_out3 : Outport  Port=5
  imag_out3 : Outport  Port=6
  real_out4 : Outport  Port=7
  imag_out4 : Outport  Port=8
  real_out5 : Outport  Port=9
  imag_out5 : Outport  Port=10
  real_out6 : Outport  Port=11
  imag_out6 : Outport  Port=12
  real_out7 : Outport  Port=13
  imag_out7 : Outport  Port=14
  real_out8 : Outport  Port=15
  imag_out8 : Outport  Port=16
  real_back_out1 : Outport  Port=17
  imag_back_out1 : Outport  Port=18
  real_back_out2 : Outport  Port=19
  imag_back_out2 : Outport  Port=20
  real_back_out3 : Outport  Port=21
  imag_back_out3 : Outport  Port=22
  real_back_out4 : Outport  Port=23
  imag_back_out4 : Outport  Port=24
  real_back_out5 : Outport  Port=25
  imag_back_out5 : Outport  Port=26
  real_back_out6 : Outport  Port=27
  imag_back_out6 : Outport  Port=28
  real_back_out7 : Outport  Port=29
  imag_back_out7 : Outport  Port=30
  real_back_out8 : Outport  Port=31
  imag_back_out8 : Outport  Port=32
  real_sum : Outport  Port=33
  imag_sum : Outport  Port=34
  wires:
  adder_tree1/1(sync_out) -> term1/1
  adder_tree2/1(sync_out) -> term2/1
  c1/1 -> adder_tree1/1(sync)
  c2/1 -> adder_tree2/1(sync)
  adder_tree1/2(dout) -> real_sum/1
  adder_tree2/2(dout) -> imag_sum/1
  real1/1 -> fir_dbl_tap1/1(a)
  imag1/1 -> fir_dbl_tap1/2(b)
  real_back8/1 -> fir_dbl_tap1/3(c)
  imag_back8/1 -> fir_dbl_tap1/4(d)
  fir_dbl_tap1/1(a_out) -> real_out1/1
  fir_dbl_tap1/2(b_out) -> imag_out1/1
  fir_dbl_tap1/3(c_out) -> real_back_out8/1
  fir_dbl_tap1/4(d_out) -> imag_back_out8/1
  fir_dbl_tap1/5(real) -> adder_tree1/2(din1)
  fir_dbl_tap1/6(imag) -> adder_tree2/2(din1)
  real2/1 -> fir_dbl_tap2/1(a)
  imag2/1 -> fir_dbl_tap2/2(b)
  real_back7/1 -> fir_dbl_tap2/3(c)
  imag_back7/1 -> fir_dbl_tap2/4(d)
  fir_dbl_tap2/1(a_out) -> real_out2/1
  fir_dbl_tap2/2(b_out) -> imag_out2/1
  fir_dbl_tap2/3(c_out) -> real_back_out7/1
  fir_dbl_tap2/4(d_out) -> imag_back_out7/1
  fir_dbl_tap2/5(real) -> adder_tree1/3(din2)
  fir_dbl_tap2/6(imag) -> adder_tree2/3(din2)
  real3/1 -> fir_dbl_tap3/1(a)
  imag3/1 -> fir_dbl_tap3/2(b)
  real_back6/1 -> fir_dbl_tap3/3(c)
  imag_back6/1 -> fir_dbl_tap3/4(d)
  fir_dbl_tap3/1(a_out) -> real_out3/1
  fir_dbl_tap3/2(b_out) -> imag_out3/1
  fir_dbl_tap3/3(c_out) -> real_back_out6/1
  fir_dbl_tap3/4(d_out) -> imag_back_out6/1
  fir_dbl_tap3/5(real) -> adder_tree1/4(din3)
  fir_dbl_tap3/6(imag) -> adder_tree2/4(din3)
  real4/1 -> fir_dbl_tap4/1(a)
  imag4/1 -> fir_dbl_tap4/2(b)
  real_back5/1 -> fir_dbl_tap4/3(c)
  imag_back5/1 -> fir_dbl_tap4/4(d)
  fir_dbl_tap4/1(a_out) -> real_out4/1
  fir_dbl_tap4/2(b_out) -> imag_out4/1
  fir_dbl_tap4/3(c_out) -> real_back_out5/1
  fir_dbl_tap4/4(d_out) -> imag_back_out5/1
  fir_dbl_tap4/5(real) -> adder_tree1/5(din4)
  fir_dbl_tap4/6(imag) -> adder_tree2/5(din4)
  real5/1 -> fir_dbl_tap5/1(a)
  imag5/1 -> fir_dbl_tap5/2(b)
  real_back4/1 -> fir_dbl_tap5/3(c)
  imag_back4/1 -> fir_dbl_tap5/4(d)
  fir_dbl_tap5/1(a_out) -> real_out5/1
  fir_dbl_tap5/2(b_out) -> imag_out5/1
  fir_dbl_tap5/3(c_out) -> real_back_out4/1
  fir_dbl_tap5/4(d_out) -> imag_back_out4/1
  fir_dbl_tap5/5(real) -> adder_tree1/6(din5)
  fir_dbl_tap5/6(imag) -> adder_tree2/6(din5)
  real6/1 -> fir_dbl_tap6/1(a)
  imag6/1 -> fir_dbl_tap6/2(b)
  real_back3/1 -> fir_dbl_tap6/3(c)
  imag_back3/1 -> fir_dbl_tap6/4(d)
  fir_dbl_tap6/1(a_out) -> real_out6/1
  fir_dbl_tap6/2(b_out) -> imag_out6/1
  fir_dbl_tap6/3(c_out) -> real_back_out3/1
  fir_dbl_tap6/4(d_out) -> imag_back_out3/1
  fir_dbl_tap6/5(real) -> adder_tree1/7(din6)
  fir_dbl_tap6/6(imag) -> adder_tree2/7(din6)
  real7/1 -> fir_dbl_tap7/1(a)
  imag7/1 -> fir_dbl_tap7/2(b)
  real_back2/1 -> fir_dbl_tap7/3(c)
  imag_back2/1 -> fir_dbl_tap7/4(d)
  fir_dbl_tap7/1(a_out) -> real_out7/1
  fir_dbl_tap7/2(b_out) -> imag_out7/1
  fir_dbl_tap7/3(c_out) -> real_back_out2/1
  fir_dbl_tap7/4(d_out) -> imag_back_out2/1
  fir_dbl_tap7/5(real) -> adder_tree1/8(din7)
  fir_dbl_tap7/6(imag) -> adder_tree2/8(din7)
  real8/1 -> fir_dbl_tap8/1(a)
  imag8/1 -> fir_dbl_tap8/2(b)
  real_back1/1 -> fir_dbl_tap8/3(c)
  imag_back1/1 -> fir_dbl_tap8/4(d)
  fir_dbl_tap8/1(a_out) -> real_out8/1
  fir_dbl_tap8/2(b_out) -> imag_out8/1
  fir_dbl_tap8/3(c_out) -> real_back_out1/1
  fir_dbl_tap8/4(d_out) -> imag_back_out1/1
  fir_dbl_tap8/5(real) -> adder_tree1/9(din8)
  fir_dbl_tap8/6(imag) -> adder_tree2/9(din8)
